simulink model "Car_14DOF_Lat_Long_Control_DATAGEN"  (R2024b)
settings: Solver=ode4  StartTime=0.0  StopTime=30  FixedStep=0.001  RelTol=1e-3
undefined symbols (not defined in the file): Ar1, Ar2, Ar3, Ar4, b, c, C_alpha, C_sigma, f, g, gradbp, Iw, Ix, Iy, Iz, k, ki, kp, kR, L, lf, lh, lr, lw, m, mR, psi0, reff, uFz, x0, xRef2s, y0, yRef2s, z0
libraries: vehdynlibviscommon x1
settings Model: Creator=sherlock2204  LastModifiedBy=sherlock2204

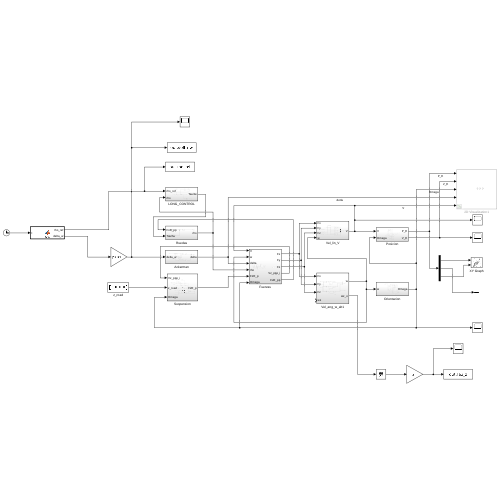
[thumbnail: Simulink's stored preview of the top-level diagram]
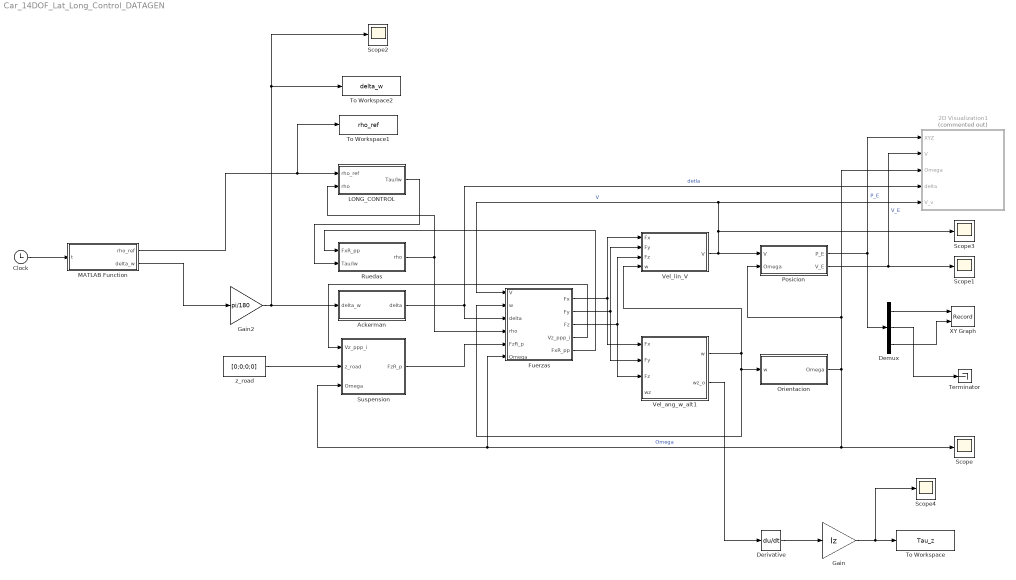
== system Car_14DOF_Lat_Long_Control_DATAGEN ==
  2D Visualization1 : Subsystem  Commented=on
      mask Display: image("visualization.JPG");
  Ackerman : Subsystem
  Clock : Clock
  Demux : Demux  Outputs=3
  Derivative : Derivative
  Fuerzas : Subsystem
  Gain : Gain  Gain=Iz
  Gain2 : Gain  Gain=pi/180
  LONG_CONTROL : Subsystem
  MATLAB Function : MATLAB Function  TreatAsAtomicUnit=on
  Orientacion : Subsystem
  Posicion : Subsystem
  Ruedas : Subsystem
  Scope{,1..4} (5 alike) : Scope
  Suspension : Subsystem
  Terminator : Terminator
  To Workspace : ToWorkspace  VariableName=Tau_z  SaveFormat=Timeseries  SampleTime=-1
  To Workspace1 : ToWorkspace  VariableName=rho_ref  SaveFormat=Timeseries  SampleTime=-1
  To Workspace2 : ToWorkspace  VariableName=delta_w  SaveFormat=Timeseries  SampleTime=-1
  Vel_ang_w_alt1 : Subsystem
  Vel_lin_V : Subsystem
  XY Graph : Record  FileSettingsInternal="{\"entries\":[{\"content\":{\"excelSettings\":{\"content\":{},\"type\":\"Streamout.ExcelSettings\"}},\"type\":\"Streamout.FileSettingStorage\",\"uuid\":\"\"}],\"packageUris\":[\"http:\\/\\/schema.mathworks.com\\/mf0\\/streamout_blocks\\/R2020a\"],\"version\":\"1.0\"}"  Layout=[1 1]  SignalsInternal="{\"entries\":[{\"content\":{\"signals\":[{\"content\":{\"blockPath\":[],\"dimensions\":[1],\"domain\":\"\",\"lineColor\":\"#edb120\",\"lineWidth\":2,\"port\":1,\"sid\":[\"\"],\"signalID\":1,\"signalName\":\"Demux:1\"},\"type\":\"RecordBlkView.Signal\",\"uuid\":\"\"},{\"content\":{\"blockPath\":[],\"dimensions\":[1],\"domain\":\"\",\"lineColor\":\"#7e2f8e\",\"lineWidth\":2,\"port\":2,\"sid\":[\"\"],\"signalID\":2,\"signalName\":\"Demux:3\"},\"type\":\"RecordBlkView.Signal\",\"uuid\":\"\"}]},\"type\":\"RecordBlkView.InputSignals\",\"uuid\":\"\"}],\"packageUris\":[\"http:\\/\\/schema.mathworks.com\\/mf0\\/streamout_blocks\\/R2020a\"],\"version\":\"1.0\"}"  VisualizationBindings="{\"xyplotplugin\":{\"info\":[{\"series\":[],\"subplotID\":1}]}}"  CompatibilityTag=XY
  z_road : Constant  Value=[0;0;0;0]
  wires:
  z_road/1 -> Suspension/2(z_road)
  Fuerzas/3(Fz) -> Vel_ang_w_alt1/3(Fz), Vel_lin_V/3(Fz)
  Vel_ang_w_alt1/1(w) -> Orientacion/1(w), Fuerzas/2(w), Vel_lin_V/4(w)
  Vel_lin_V/1(V) -> Posicion/1(V), Scope3/1, 2D Visualization1/5(V_v), Fuerzas/1(V)  "V"
  Suspension/1(FzR_p) -> Fuerzas/5(FzR_p)
  Fuerzas/4(Vz_ppp_i) -> Suspension/1(Vz_ppp_i)
  Ackerman/1(delta) -> 2D Visualization1/4(delta), Fuerzas/3(delta)  "detla"
  Demux/1 -> XY Graph/1
  Demux/3 -> XY Graph/2
  Demux/2 -> Terminator/1
  Fuerzas/1(Fx) -> Vel_ang_w_alt1/1(Fx), Vel_lin_V/1(Fx)
  Fuerzas/2(Fy) -> Vel_ang_w_alt1/2(Fy), Vel_lin_V/2(Fy)
  Orientacion/1(Omega) -> 2D Visualization1/3(Omega), Posicion/2(Omega), Scope/1, Fuerzas/6(Omega), Suspension/3(Omega)  "Omega"
  Posicion/2(V_E) -> Scope1/1, 2D Visualization1/2(V)  "V_E"
  Posicion/1(P_E) -> Demux/1, 2D Visualization1/1(XYZ)  "P_E"
  Fuerzas/5(FxR_pp) -> Ruedas/1(FxR_pp)
  Ruedas/1(rho) -> Fuerzas/4(rho), LONG_CONTROL/2(rho)
  MATLAB Function/1(rho_ref) -> To Workspace1/1, LONG_CONTROL/1(rho_ref)
  LONG_CONTROL/1(Tau/Iw) -> Ruedas/2(Tau/Iw)
  Gain2/1 -> To Workspace2/1, Scope2/1, Ackerman/1(delta_w)
  Clock/1 -> MATLAB Function/1(t)
  Vel_ang_w_alt1/2(wz_o) -> Derivative/1
  Derivative/1 -> Gain/1
  Gain/1 -> Scope4/1, To Workspace/1
  MATLAB Function/2(delta_w) -> Gain2/1

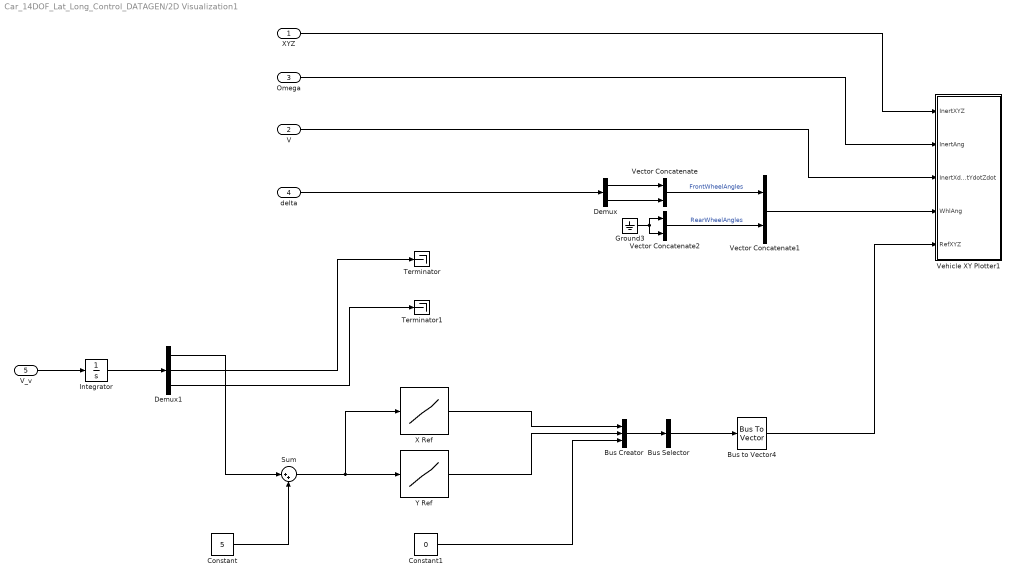
== system Car_14DOF_Lat_Long_Control_DATAGEN/2D Visualization1 ==
  XYZ : Inport
  V : Inport  Port=2
  Omega : Inport  Port=3
  delta : Inport  Port=4
  V_v : Inport  Port=5
  Bus Creator : BusCreator  Inputs=3
  Bus Selector : BusSelector  OutputSignals=signal1,signal2,signal3  OutputAsBus=on
  Bus to Vector4 : BusToVector
  Constant : Constant  Value=5
  Constant1 : Constant  Value=0
  Demux : Demux  Outputs=2
  Demux1 : Demux  Outputs=3
  Ground3 : Ground
  Integrator : Integrator
  Sum : Sum  Inputs=|++
  Terminator : Terminator
  Terminator1 : Terminator
  Vector Concatenate : Concatenate
  Vector Concatenate1 : Concatenate
  Vector Concatenate2 : Concatenate
  Vehicle XY Plotter1 : Subsystem  mask(Vehicle XY Plotter){extRef=on, extStats=off, extTireF=off, a=lf, b=lr, w=c, figBorder=10, bufferSize=1024, velNorm=5, tireFNorm=1000, pltDT=0.2}
      mask prompts: extRef "Plot path reference, extRef"; extStats "Display speed, RPM and Gear"; extTireF "Display tire forces"; a "Distance to front axle from CG, a [m]:"; b "Distance to rear axle from CG, b [m]:"; w "Track width, w [m]:"; figBorder "Distance to figure borders, figBorder [m]:"; bufferSize "Path buffer sampe size, bufferSize []:"; velNorm "Velocity vector scaling, velNorm [m*s/m]:"; tireFNorm "Tire force vector scaling, tireFNorm [m/N]:"; pltDT "Plot update rate, pltDT [s]:"
      mask help:
      | This block will display a MATLAB figure which indicates the vehicle path, current position and heading velocity.
      | An optional path reference is also provided.
      mask init:
      | block = gcb;
      | if autoblkschecksimstopped(block)
      |     ParamNames = {'extRef';'extStats';'extTireF';'extTireF'};
      |     PortNames = {'RefXYZ';'Stats';'TireFx';'TireFy'};
      |     for idx=1:length(PortNames)
      |         InportOption  = {'built-in/Ground', [PortNames{idx}, ' Ground'];...
      |             'built-in/Inport',PortNames{idx}};
      |         if ~strcmp(get_param(block,ParamNames{idx}),'on')
      |             NewBlkHdl = autoblksreplaceblock(block, InportOption, 1);
      |             set_param(NewBlkHdl, 'ShowName', 'off');
      |         else
      |             autoblksreplaceblock(block, InportOption, 2);
      |         end
      |     end
      |     InportNames = {'InertXYZ';'InertAng';'InertXdotYdotZdot';'WhlAng';'RefXYZ';'Stats';'TireFx';'TireFy'};
      |     FoundNames = get_param(find_system(block, 'LookUnderMasks', 'all', 'SearchDepth', 1, 'FollowLinks', 'on', 'BlockType', 'Inport'), 'Name');
      |     [~,PortI] = intersect(InportNames, FoundNames);
      |     PortI = sort(PortI);
      |     for idx = 1:length(PortI)
      |         set_param([block, '/', InportNames{PortI(idx)}], 'Port', num2str(idx));
      |     end
      | end
      mask TypeOptions a: Vehicle XY Plotter/a
      mask TypeOptions b: Vehicle XY Plotter/b
      mask TypeOptions w: Vehicle XY Plotter/w
      mask TypeOptions figBorder: Vehicle XY Plotter/figBorder
      mask TypeOptions bufferSize: Vehicle XY Plotter/bufferSize
      mask TypeOptions velNorm: Vehicle XY Plotter/velNorm
      mask TypeOptions tireFNorm: Vehicle XY Plotter/tireFNorm
      mask DialogControl Container3 Prompt: Plot and Display Options
  X Ref : Lookup_n-D  NumberOfTableDimensions=1  BreakpointsForDimension1=gradbp  Table=xRef2s  InternalRulePriority=Speed  RndMeth=Simplest
  Y Ref : Lookup_n-D  NumberOfTableDimensions=1  BreakpointsForDimension1=gradbp  Table=yRef2s  InternalRulePriority=Speed  RndMeth=Simplest
  wires:
  Omega/1 -> Vehicle XY Plotter1/2(InertAng)
  XYZ/1 -> Vehicle XY Plotter1/1(InertXYZ)
  V/1 -> Vehicle XY Plotter1/3(InertXdotYdotZdot)
  Vector Concatenate2/1 -> Vector Concatenate1/2  "RearWheelAngles"
  Vector Concatenate/1 -> Vector Concatenate1/1  "FrontWheelAngles"
  Ground3/1 -> Vector Concatenate2/2, Vector Concatenate2/1
  Vector Concatenate1/1 -> Vehicle XY Plotter1/4(WhlAng)
  delta/1 -> Demux/1
  Demux/1 -> Vector Concatenate/1
  Demux/2 -> Vector Concatenate/2
  Bus Creator/1 -> Bus Selector/1
  Y Ref/1 -> Bus Creator/2
  Bus Selector/1 -> Bus to Vector4/1
  Demux1/3 -> Terminator1/1
  X Ref/1 -> Bus Creator/1
  Constant1/1 -> Bus Creator/3
  Bus to Vector4/1 -> Vehicle XY Plotter1/5(RefXYZ)
  Demux1/2 -> Terminator/1
  V_v/1 -> Integrator/1
  Integrator/1 -> Demux1/1
  Demux1/1 -> Sum/1
  Sum/1 -> X Ref/1, Y Ref/1
  Constant/1 -> Sum/2

== system Car_14DOF_Lat_Long_Control_DATAGEN/Ackerman ==
  delta_w : Inport
  Atan : Trigonometry  Operator=atan
  Atan1 : Trigonometry  Operator=atan
  Constant : Constant  Value=L
  Divide : Product  Inputs=*/
  Divide1 : Product  Inputs=*/
  Gain : Gain  Gain=L
  Gain1 : Gain  Gain=lw
  Mux : Mux  Inputs=2
  Sum : Sum  Inputs=++|
  Sum1 : Sum  Inputs=-+|
  Tan : Trigonometry  Operator=tan
  delta : Outport
  wires:
  Mux/1 -> delta/1
  delta_w/1 -> Tan/1
  Tan/1 -> Gain/1, Gain1/1
  Gain/1 -> Divide1/1, Divide/1
  Divide/1 -> Atan/1
  Constant/1 -> Sum/2, Sum1/2
  Gain1/1 -> Sum/1, Sum1/1
  Sum/1 -> Divide/2
  Sum1/1 -> Divide1/2
  Divide1/1 -> Atan1/1
  Atan/1 -> Mux/1
  Atan1/1 -> Mux/2

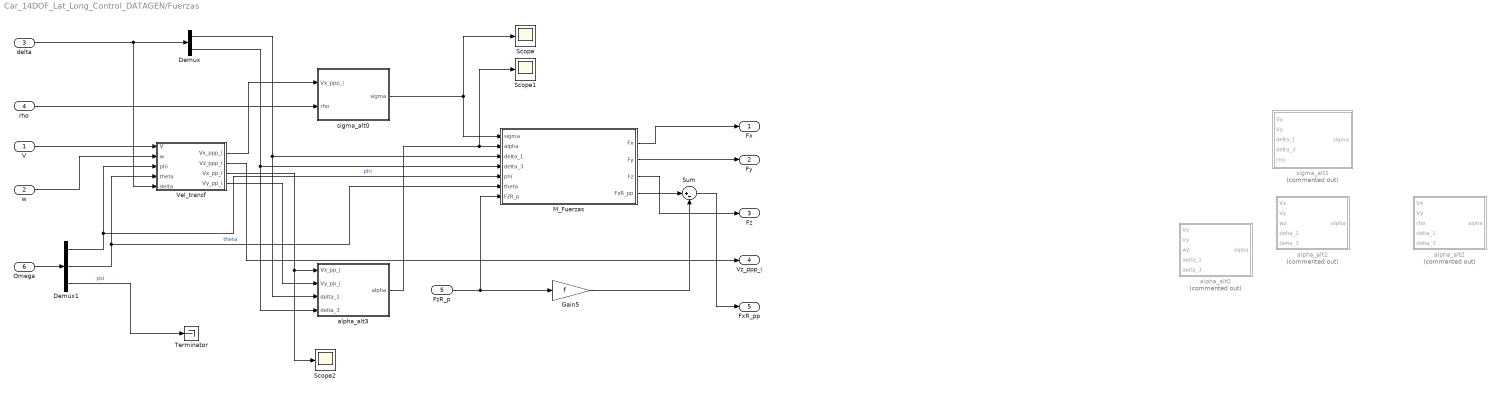
== system Car_14DOF_Lat_Long_Control_DATAGEN/Fuerzas ==
  V : Inport
  w : Inport  Port=2
  delta : Inport  Port=3
  rho : Inport  Port=4
  FzR_p : Inport  Port=5
  Omega : Inport  Port=6
  Demux : Demux  Outputs=2
  Demux1 : Demux  Outputs=3
  Gain5 : Gain  Gain=f
  M_Fuerzas : Subsystem
  Scope : Scope
  Scope1 : Scope
  Scope2 : Scope
  Sum : Sum  Inputs=|+-
  Terminator : Terminator
  Vel_transf : Subsystem
  alpha_alt0 : Subsystem  Commented=on
  alpha_alt1 : Subsystem  Commented=on
  alpha_alt2 : Subsystem  Commented=on
  alpha_alt3 : Subsystem
  sigma_alt0 : Subsystem
  sigma_alt1 : Subsystem  Commented=on
  Fx : Outport
  Fy : Outport  Port=2
  Fz : Outport  Port=3
  Vz_ppp_i : Outport  Port=4
  FxR_pp : Outport  Port=5
  wires:
  V/1 -> Vel_transf/1(V)
  w/1 -> Vel_transf/2(w)
  Demux1/1 -> Vel_transf/3(phi), M_Fuerzas/5(phi)  "phi"
  Demux1/2 -> M_Fuerzas/6(theta), Vel_transf/4(theta)  "theta"
  M_Fuerzas/2(Fy) -> Fy/1
  M_Fuerzas/3(Fz) -> Fz/1
  delta/1 -> Vel_transf/5(delta), Demux/1
  Demux/2 -> alpha_alt3/4(delta_3), M_Fuerzas/4(delta_3)
  Demux/1 -> M_Fuerzas/3(delta_1), alpha_alt3/3(delta_1)
  rho/1 -> sigma_alt0/2(rho)
  Vel_transf/1(Vx_ppp_i) -> sigma_alt0/1(Vx_ppp_i)
  sigma_alt0/1(sigma) -> M_Fuerzas/1(sigma), Scope/1
  alpha_alt3/1(alpha) -> M_Fuerzas/2(alpha), Scope1/1
  FzR_p/1 -> Gain5/1, M_Fuerzas/7(FzR_p)
  Vel_transf/2(Vz_ppp_i) -> Vz_ppp_i/1
  Vel_transf/3(Vx_pp_i) -> Scope2/1, alpha_alt3/1(Vx_pp_i)
  Vel_transf/4(Vy_pp_i) -> alpha_alt3/2(Vy_pp_i)
  Omega/1 -> Demux1/1
  Demux1/3 -> Terminator/1  "psi"
  M_Fuerzas/1(Fx) -> Fx/1
  M_Fuerzas/4(FxR_pp) -> Sum/1
  Sum/1 -> FxR_pp/1
  Gain5/1 -> Sum/2

== system Car_14DOF_Lat_Long_Control_DATAGEN/LONG_CONTROL ==
  rho_ref : Inport
  rho : Inport  Port=2
  Add : Sum  Inputs=+++
  Add1 : Sum  Inputs=++++
  Demux : Demux
  Derivative : Derivative
  Gain : Gain  Gain=[1;1;1;1]
  Gain1 : Gain  Gain=Iw
  Gain2 : Gain  Gain=-ki
  Gain3 : Gain  Gain=-kp
  Integrator5 : Integrator
  Scope : Scope
  Scope1 : Scope
  Sum1 : Sum  Inputs=|-+
  Tau/Iw : Outport
  wires:
  Gain/1 -> Sum1/1, Derivative/1
  Add/1 -> Gain1/1, Tau/Iw/1  "u=Tau/Iw"
  Integrator5/1 -> Gain2/1  "Ie_rho"
  Gain3/1 -> Add/2
  Sum1/1 -> Integrator5/1, Gain3/1  "e_rho"
  Gain2/1 -> Add/1  "-z"
  Derivative/1 -> Add/3  "Drho_ref"
  rho_ref/1 -> Gain/1
  rho/1 -> Scope1/1, Sum1/2
  Gain1/1 -> Demux/1
  Demux/1 -> Add1/1
  Demux/2 -> Add1/2
  Demux/3 -> Add1/3
  Demux/4 -> Add1/4
  Add1/1 -> Scope/1

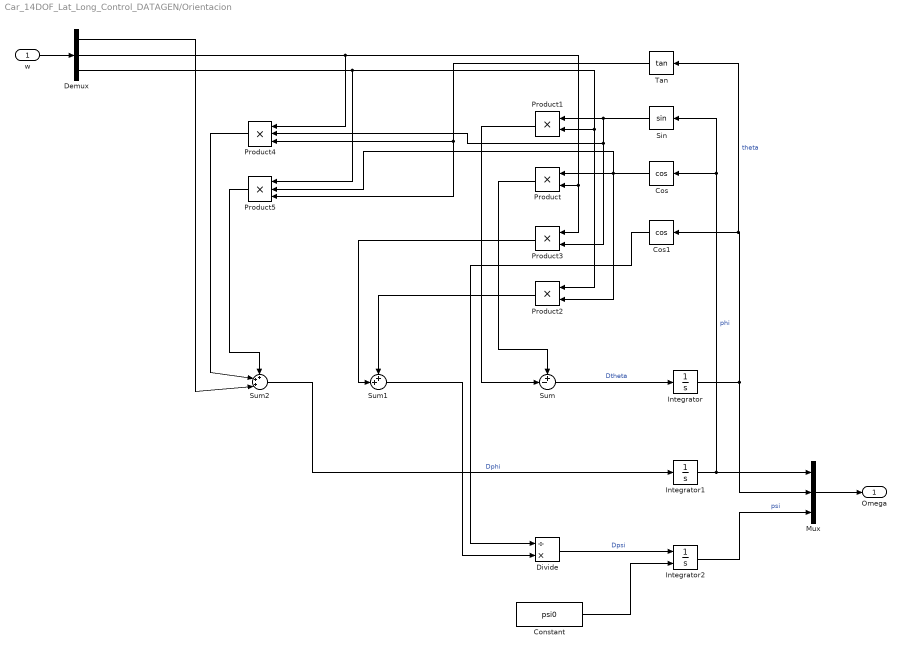
== system Car_14DOF_Lat_Long_Control_DATAGEN/Orientacion ==
  w : Inport
  Constant : Constant  Value=psi0
  Cos : Trigonometry  Operator=cos
  Cos1 : Trigonometry  Operator=cos
  Demux : Demux  Outputs=3
  Divide : Product  Inputs=/*
  Integrator : Integrator
  Integrator1 : Integrator
  Integrator2 : Integrator  InitialConditionSource=external
  Mux : Mux  Inputs=3
  Product{,1..3} (4 alike) : Product
  Product4 : Product  Inputs=3
  Product5 : Product  Inputs=3
  Sin : Trigonometry
  Sum : Sum  Inputs=+-|
  Sum1 : Sum  Inputs=++|
  Sum2 : Sum  Inputs=+++|
  Tan : Trigonometry  Operator=tan
  Omega : Outport
  wires:
  w/1 -> Demux/1
  Integrator/1 -> Mux/2, Tan/1, Cos1/1  "theta"
  Integrator2/1 -> Mux/3  "psi"
  Sin/1 -> Product4/2, Product3/2, Product1/1
  Cos/1 -> Product5/2, Product2/2, Product/1
  Demux/2 -> Product4/1, Product3/1, Product/2
  Demux/3 -> Product5/1, Product2/1, Product1/2
  Product/1 -> Sum/1
  Product1/1 -> Sum/2
  Sum/1 -> Integrator/1  "Dtheta"
  Integrator1/1 -> Sin/1, Cos/1, Mux/1  "phi"
  Product2/1 -> Sum1/1
  Product3/1 -> Sum1/2
  Divide/1 -> Integrator2/1  "Dpsi"
  Sum1/1 -> Divide/2
  Cos1/1 -> Divide/1
  Tan/1 -> Product4/3, Product5/3
  Sum2/1 -> Integrator1/1  "Dphi"
  Product5/1 -> Sum2/1
  Product4/1 -> Sum2/2
  Demux/1 -> Sum2/3
  Mux/1 -> Omega/1
  Constant/1 -> Integrator2/2

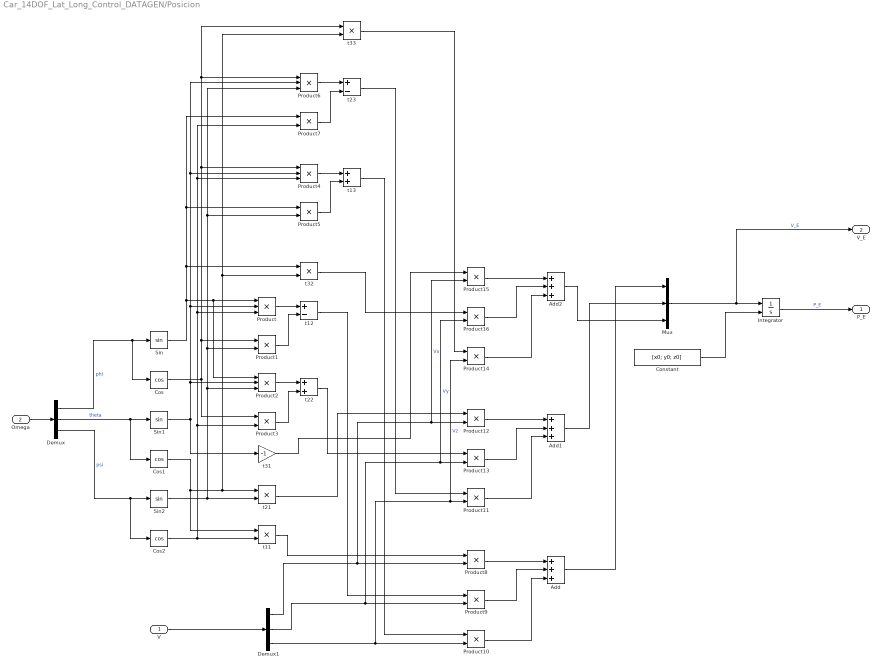
== system Car_14DOF_Lat_Long_Control_DATAGEN/Posicion ==
  V : Inport
  Omega : Inport  Port=2
  Add : Sum  Inputs=+++
  Add1 : Sum  Inputs=+++
  Add2 : Sum  Inputs=+++
  Constant : Constant  Value=[x0; y0; z0]
  Cos : Trigonometry  Operator=cos
  Cos1 : Trigonometry  Operator=cos
  Cos2 : Trigonometry  Operator=cos
  Demux : Demux  Outputs=3
  Demux1 : Demux  Outputs=3
  Integrator : Integrator  InitialConditionSource=external
  Mux : Mux  Inputs=3
  Product{,2,4,6} (4 alike) : Product  Inputs=3
  Product{1,3,5,7..16} (13 alike) : Product
  Sin : Trigonometry
  Sin1 : Trigonometry
  Sin2 : Trigonometry
  t{11,21,32..33} (4 alike) : Product
  t12 : Sum  Inputs=+-
  t13 : Sum
  t22 : Sum
  t23 : Sum  Inputs=+-
  t31 : Gain  Gain=-1
  P_E : Outport
  V_E : Outport  Port=2
  wires:
  Demux/1 -> Cos/1, Sin/1  "phi"
  Demux/2 -> Cos1/1, Sin1/1  "theta"
  Demux/3 -> Cos2/1, Sin2/1  "psi"
  Omega/1 -> Demux/1
  Cos2/1 -> Product7/2, Product4/3, Product/3, Product3/2, t11/2
  Cos1/1 -> t21/1, t33/2, t32/2, t11/1
  Sin2/1 -> Product6/3, Product5/2, Product1/2, Product2/3, t21/2
  Sin1/1 -> Product6/2, Product4/2, Product/2, Product2/2, t31/1
  Sin/1 -> Product7/1, Product5/1, t32/1, Product2/1, Product/1
  Cos/1 -> t33/1, Product6/1, Product4/1, Product1/1, Product3/1
  Product/1 -> t12/1
  Product1/1 -> t12/2
  Product3/1 -> t22/2
  Product2/1 -> t22/1
  Product5/1 -> t13/2
  Product4/1 -> t13/1
  Product6/1 -> t23/1
  Product7/1 -> t23/2
  V/1 -> Demux1/1
  Demux1/1 -> Product15/2, Product12/2, Product8/2  "Vx"
  Demux1/3 -> Product10/2, Product14/2, Product11/2  "Vz"
  Demux1/2 -> Product9/2, Product16/2, Product13/2  "Vy"
  t11/1 -> Product8/1
  t12/1 -> Product9/1
  t13/1 -> Product10/1
  Product8/1 -> Add/1
  Product9/1 -> Add/2
  Product10/1 -> Add/3
  Product13/1 -> Add1/2
  Product12/1 -> Add1/1
  Product11/1 -> Add1/3
  t21/1 -> Product12/1
  t22/1 -> Product13/1
  t23/1 -> Product11/1
  Product15/1 -> Add2/1
  Product16/1 -> Add2/2
  Product14/1 -> Add2/3
  t31/1 -> Product15/1
  t32/1 -> Product16/1
  t33/1 -> Product14/1
  Add/1 -> Mux/1
  Add1/1 -> Mux/2
  Add2/1 -> Mux/3
  Mux/1 -> V_E/1, Integrator/1  "V_E"
  Integrator/1 -> P_E/1  "P_E"
  Constant/1 -> Integrator/2

== system Car_14DOF_Lat_Long_Control_DATAGEN/Ruedas ==
  FxR_pp : Inport
  Tau/Iw : Inport  Port=2
  Gain : Gain  Gain=1/Iw
  Gain13 : Gain  Gain=-reff/Iw
  Integrator4 : Integrator
  Sum : Sum  Inputs=|++
  rho : Outport
  wires:
  FxR_pp/1 -> Gain13/1
  Tau/Iw/1 -> Gain/1  "u=Tau/Iw"
  Sum/1 -> Integrator4/1  "Drho"
  Integrator4/1 -> rho/1
  Gain13/1 -> Sum/2  "EPS(t)"
  Gain/1 -> Sum/1  "Tau"

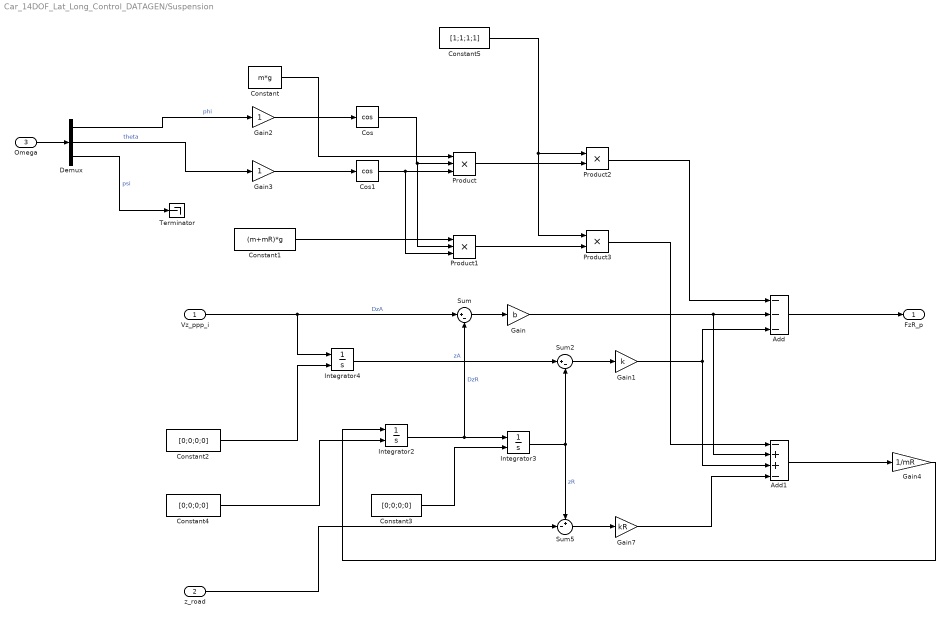
== system Car_14DOF_Lat_Long_Control_DATAGEN/Suspension ==
  Vz_ppp_i : Inport
  z_road : Inport  Port=2
  Omega : Inport  Port=3
  Add : Sum  Inputs=---
  Add1 : Sum  Inputs=-++-
  Constant : Constant  Value=m*g
  Constant1 : Constant  Value=(m+mR)*g
  Constant2 : Constant  Value=[0;0;0;0]
  Constant3 : Constant  Value=[0;0;0;0]
  Constant4 : Constant  Value=[0;0;0;0]
  Constant5 : Constant  Value=[1;1;1;1]
  Cos : Trigonometry  Operator=cos
  Cos1 : Trigonometry  Operator=cos
  Demux : Demux  Outputs=3
  Gain : Gain  Gain=b
  Gain1 : Gain  Gain=k
  Gain2 : Gain
  Gain3 : Gain
  Gain4 : Gain  Gain=1/mR
  Gain7 : Gain  Gain=kR
  Integrator2 : Integrator  InitialConditionSource=external
  Integrator3 : Integrator  InitialConditionSource=external
  Integrator4 : Integrator  InitialConditionSource=external
  Product : Product  Inputs=3
  Product1 : Product  Inputs=3
  Product2 : Product
  Product3 : Product
  Sum : Sum  Inputs=|+-
  Sum2 : Sum  Inputs=|+-
  Sum5 : Sum  Inputs=+-|
  Terminator : Terminator
  FzR_p : Outport
  wires:
  Sum/1 -> Gain/1
  Integrator3/1 -> Sum2/2, Sum5/1  "zR"
  Sum2/1 -> Gain1/1
  Add/1 -> FzR_p/1
  Add1/1 -> Gain4/1
  Gain/1 -> Add1/2, Add/2
  Integrator2/1 -> Integrator3/1, Sum/2  "DzR"
  Gain1/1 -> Add/3, Add1/3
  Sum5/1 -> Gain7/1
  Gain7/1 -> Add1/4
  Gain4/1 -> Integrator2/1
  Constant4/1 -> Integrator2/2
  Constant3/1 -> Integrator3/2
  z_road/1 -> Sum5/2
  Cos1/1 -> Product1/3, Product/3
  Cos/1 -> Product1/2, Product/2
  Constant/1 -> Product/1
  Constant1/1 -> Product1/1
  Vz_ppp_i/1 -> Integrator4/1, Sum/1  "DzA"
  Integrator4/1 -> Sum2/1  "zA"
  Constant2/1 -> Integrator4/2
  Product/1 -> Product2/2
  Constant5/1 -> Product3/1, Product2/1
  Product1/1 -> Product3/2
  Demux/1 -> Gain2/1  "phi"
  Demux/2 -> Gain3/1  "theta"
  Product2/1 -> Add/1
  Product3/1 -> Add1/1
  Gain2/1 -> Cos/1
  Gain3/1 -> Cos1/1
  Omega/1 -> Demux/1
  Demux/3 -> Terminator/1  "psi"

== system Car_14DOF_Lat_Long_Control_DATAGEN/Vel_ang_w_alt1 ==
  Fx : Inport
  Fy : Inport  Port=2
  Fz : Inport  Port=3
  wz : Inport  Port=4
  Integrator : Integrator  InitialConditionSource=external
  Integrator1 : Integrator  InitialConditionSource=external
  Integrator2 : Integrator  InitialConditionSource=external
  Multiply : Gain  Gain=(1/Ix)*[c c -c -c lh lh lh lh]  Multiplication=Matrix(K*u) (u vector)
  Multiply1 : Gain  Gain=(1/Iy)*[-lh -lh -lh -lh -lf lr -lf lr]  Multiplication=Matrix(K*u) (u vector)
  Multiply2 : Gain  Gain=(1/Iz)*[lf -lr lf -lr -c -c c c]  Multiplication=Matrix(K*u) (u vector)
  Mux : Mux  Inputs=3
  Vector Concatenate : Concatenate
  Vector Concatenate1 : Concatenate
  Vector Concatenate2 : Concatenate
  wx0 : Constant  Value=0
  wy0 : Constant  Value=0
  wz0 : Constant  Value=0
  w : Outport
  wz_o : Outport  Port=2
  wires:
  wx0/1 -> Integrator/2
  wy0/1 -> Integrator1/2
  Mux/1 -> w/1
  wz0/1 -> Integrator2/2
  Integrator/1 -> Mux/1  "wx"
  Fz/1 -> Vector Concatenate/1, Vector Concatenate1/2
  Fy/1 -> Vector Concatenate/2, Vector Concatenate2/1
  Vector Concatenate/1 -> Multiply/1
  Multiply1/1 -> Integrator1/1
  Vector Concatenate1/1 -> Multiply1/1
  Fx/1 -> Vector Concatenate2/2, Vector Concatenate1/1
  Integrator1/1 -> Mux/2  "wy"
  Vector Concatenate2/1 -> Multiply2/1
  Integrator2/1 -> Mux/3, wz_o/1  "wz"
  Multiply/1 -> Integrator/1
  Multiply2/1 -> Integrator2/1

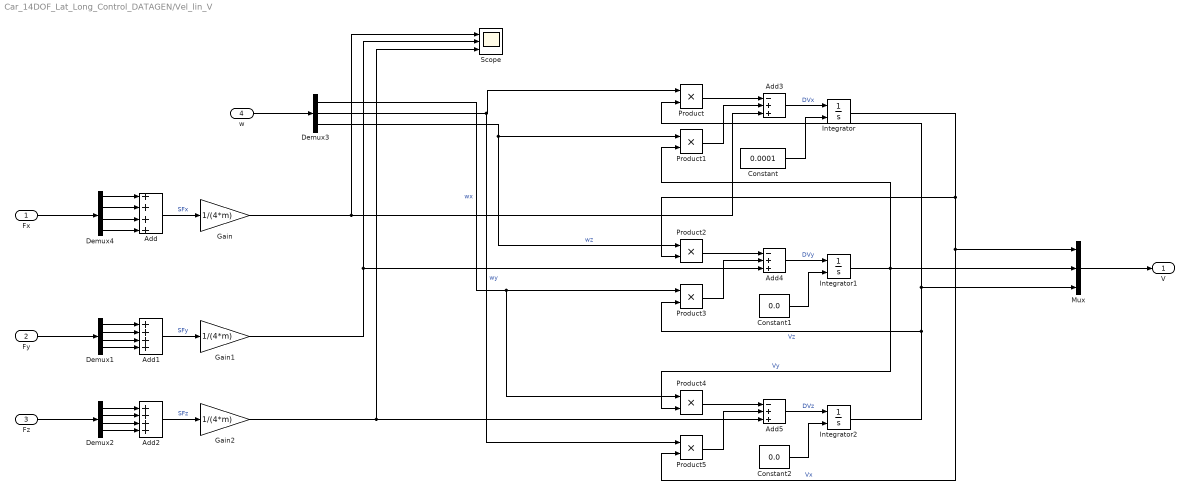
== system Car_14DOF_Lat_Long_Control_DATAGEN/Vel_lin_V ==
  Fx : Inport
  Fy : Inport  Port=2
  Fz : Inport  Port=3
  w : Inport  Port=4
  Add : Sum  Inputs=++++
  Add1 : Sum  Inputs=++++
  Add2 : Sum  Inputs=++++
  Add3 : Sum  Inputs=-++
  Add4 : Sum  Inputs=-++
  Add5 : Sum  Inputs=-++
  Constant : Constant  Value=0.0001  SampleTime=0.001
  Constant1 : Constant  Value=0.0
  Constant2 : Constant  Value=0.0
  Demux1 : Demux
  Demux2 : Demux
  Demux3 : Demux  Outputs=3
  Demux4 : Demux
  Gain : Gain  Gain=1/(4*m)
  Gain1 : Gain  Gain=1/(4*m)
  Gain2 : Gain  Gain=1/(4*m)
  Integrator : Integrator  InitialConditionSource=external  UpperSaturationLimit=27.7778  LowerSaturationLimit=-27.7778  AbsoluteTolerance=10
  Integrator1 : Integrator  InitialConditionSource=external
  Integrator2 : Integrator  InitialConditionSource=external
  Mux : Mux  Inputs=3
  Product{,1..5} (6 alike) : Product
  Scope : Scope  NumInputPorts=3
  V : Outport
  wires:
  Fy/1 -> Demux1/1
  Demux1/1 -> Add1/1
  Demux1/2 -> Add1/2
  Demux1/3 -> Add1/3
  Demux1/4 -> Add1/4
  Demux2/1 -> Add2/1
  Fz/1 -> Demux2/1
  Demux2/2 -> Add2/2
  Demux2/4 -> Add2/4
  Demux2/3 -> Add2/3
  w/1 -> Demux3/1
  Add/1 -> Gain/1  "SFx"
  Add1/1 -> Gain1/1  "SFy"
  Add2/1 -> Gain2/1  "SFz"
  Add3/1 -> Integrator/1  "DVx"
  Product1/1 -> Add3/2
  Product/1 -> Add3/1
  Demux3/3 -> Product2/1, Product1/1  "wz"
  Demux3/2 -> Product5/1, Product/1  "wy"
  Product2/1 -> Add4/1
  Add4/1 -> Integrator1/1  "DVy"
  Product3/1 -> Add4/2
  Add5/1 -> Integrator2/1  "DVz"
  Product4/1 -> Add5/1
  Product5/1 -> Add5/2
  Demux3/1 -> Product4/1, Product3/1  "wx"
  Integrator1/1 -> Mux/2, Product1/2, Product4/2  "Vy"
  Integrator2/1 -> Product3/2, Mux/3, Product/2  "Vz"
  Integrator/1 -> Mux/1, Product5/2, Product2/2  "Vx"
  Mux/1 -> V/1
  Demux4/1 -> Add/1
  Demux4/4 -> Add/4
  Demux4/2 -> Add/2
  Demux4/3 -> Add/3
  Fx/1 -> Demux4/1
  Constant/1 -> Integrator/2
  Constant1/1 -> Integrator1/2
  Constant2/1 -> Integrator2/2
  Gain/1 -> Scope/1, Add3/3
  Gain1/1 -> Scope/2, Add4/3
  Gain2/1 -> Scope/3, Add5/3

== system Car_14DOF_Lat_Long_Control_DATAGEN/2D Visualization1/Vehicle XY Plotter1 ==
  InertXYZ : Inport
  InertAng : Inport  Port=2
  InertXdotYdotZdot : Inport  Port=3
  WhlAng : Inport  Port=4
  RefXYZ : Inport  Port=5
  Data Type Conversion : DataTypeConversion  OutDataTypeStr=double  SaturateOnIntegerOverflow=off  RndMeth=Floor
  Rate Transition{1..7} (7 alike) : RateTransition  Deterministic=off  OutPortSampleTime=pltDT
  Reshape : Reshape  OutputDimensionality=Row vector (2-D)
  Reshape1 : Reshape  OutputDimensionality=Row vector (2-D)
  Stats Ground : Ground
  TireFx Ground : Ground
  TireFy Ground : Ground
  Vector Concatenate : Concatenate  Mode=Multidimensional array
  Vehicle XY Plotter : vehdynlibviscommon/Vehicle XY Plotter  w=w  a=a  b=b  figBorder=figBorder  bufferSize=bufferSize  extStats=off  extTireF=off
  wires:
  Stats Ground/1 -> Data Type Conversion/1
  InertAng/1 -> Rate Transition2/1  "InertCGDisp"
  InertXdotYdotZdot/1 -> Rate Transition4/1  "InertCGVel"
  InertXYZ/1 -> Rate Transition1/1  "InertCGDisp"
  WhlAng/1 -> Rate Transition5/1  "WhlAng"
  Rate Transition3/1 -> Vehicle XY Plotter/5
  Rate Transition1/1 -> Vehicle XY Plotter/1
  Rate Transition2/1 -> Vehicle XY Plotter/2
  Rate Transition4/1 -> Vehicle XY Plotter/3
  Rate Transition5/1 -> Vehicle XY Plotter/4
  Rate Transition6/1 -> ?
  Data Type Conversion/1 -> Rate Transition6/1
  Rate Transition7/1 -> ?
  Reshape/1 -> Vector Concatenate/1
  Reshape1/1 -> Vector Concatenate/2
  Vector Concatenate/1 -> Rate Transition7/1
  TireFx Ground/1 -> Reshape/1
  TireFy Ground/1 -> Reshape1/1
  RefXYZ/1 -> Rate Transition3/1

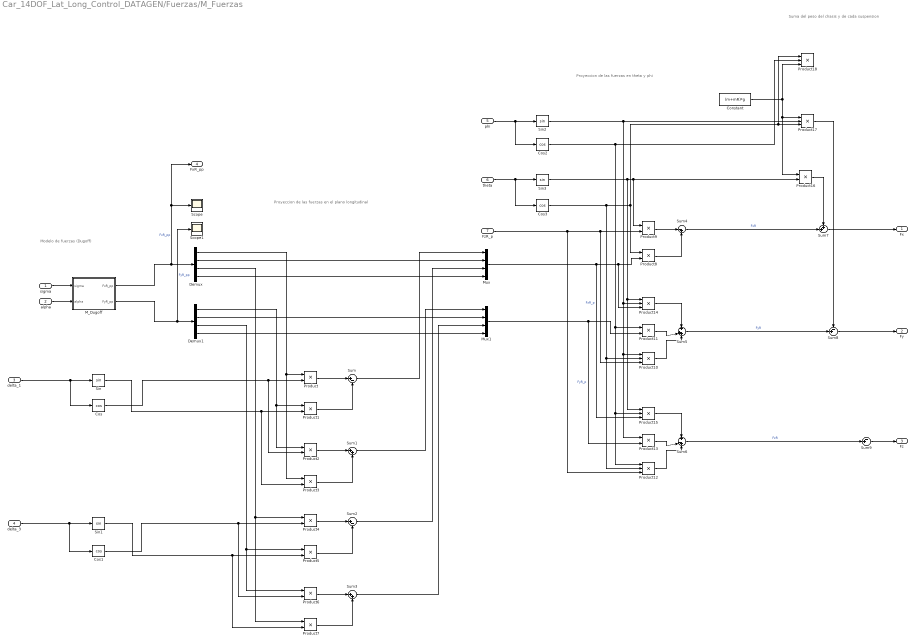
== system Car_14DOF_Lat_Long_Control_DATAGEN/Fuerzas/M_Fuerzas ==
  note: Modelo de fuerzas (Dugoff)
  note: Suma del peso del chasis
      | y de cada suspension
  note: Proyeccion de las fuerzas en theta y phi
  note: Proyeccion de las fuerzas en el plano longitudinal
  sigma : Inport
  alpha : Inport  Port=2
  delta_1 : Inport  Port=3
  delta_3 : Inport  Port=4
  phi : Inport  Port=5
  theta : Inport  Port=6
  FzR_p : Inport  Port=7
  Constant : Constant  Value=(m+mR)*g
  Cos{,1..3} (4 alike) : Trigonometry  Operator=cos
  Demux : Demux
  Demux1 : Demux
  M_Dugoff : Subsystem
  Mux : Mux
  Mux1 : Mux
  Product{,1..9,11,13,16} (13 alike) : Product
  Product{10,12,14..15,17..18} (6 alike) : Product  Inputs=3
  Scope : Scope
  Scope1 : Scope
  Sin{,1..3} (4 alike) : Trigonometry
  Sum : Sum  Inputs=|+-
  Sum1 : Sum  Inputs=|++
  Sum2 : Sum  Inputs=|+-
  Sum3 : Sum  Inputs=|++
  Sum4 : Sum  Inputs=|-+
  Sum5 : Sum  Inputs=+|++
  Sum6 : Sum  Inputs=+|-+
  Sum7 : Sum  Inputs=++|
  Sum8 : Sum  Inputs=-+|
  Sum9 : Sum  Inputs=-+|
  Fx : Outport
  Fy : Outport  Port=2
  Fz : Outport  Port=3
  FxR_pp : Outport  Port=4
  wires:
  M_Dugoff/2(FyR_pp) -> Scope1/1, Demux1/1  "FyR_pp"
  Demux/2 -> Mux/2
  Demux/4 -> Mux/4
  Demux1/2 -> Mux1/2
  Demux1/4 -> Mux1/4
  Demux/1 -> Product3/1, Product/1
  Cos/1 -> Product2/2, Product/2
  Product/1 -> Sum/1
  Sin/1 -> Product3/2, Product1/2
  Demux1/1 -> Product2/1, Product1/1
  Product1/1 -> Sum/2
  Sum/1 -> Mux/1
  Product2/1 -> Sum1/1
  Product3/1 -> Sum1/2
  Sum1/1 -> Mux1/1
  Product6/1 -> Sum3/1
  Product7/1 -> Sum3/2
  Product5/1 -> Sum2/2
  Product4/1 -> Sum2/1
  Demux/3 -> Product7/1, Product4/1
  Demux1/3 -> Product6/1, Product5/1
  Cos1/1 -> Product6/2, Product4/2
  Sin1/1 -> Product7/2, Product5/2
  Sum2/1 -> Mux/3
  Sum3/1 -> Mux1/3
  Mux/1 -> Product15/3, Product14/3, Product8/2  "FxR_p"
  FzR_p/1 -> Product12/3, Product9/2, Product10/3
  Cos3/1 -> Product12/2, Product10/2, Product18/1, Product17/3, Product8/1
  Sin3/1 -> Product15/1, Product14/1, Product9/1, Product16/2
  Product9/1 -> Sum4/1
  Product8/1 -> Sum4/2
  Product10/1 -> Sum5/3
  Sum5/1 -> Sum8/2  "FyR"
  Product11/1 -> Sum5/2
  Product13/1 -> Sum6/2
  Product12/1 -> Sum6/3
  Sum6/1 -> Sum9/2  "FzR"
  Product14/1 -> Sum5/1
  Sin2/1 -> Product17/2, Product13/1, Product10/1, Product14/2
  Mux1/1 -> Product11/2, Product13/2  "FyR_p"
  Cos2/1 -> Product18/2, Product11/1, Product12/1, Product15/2
  Product15/1 -> Sum6/1
  Constant/1 -> Product18/3, Product16/1, Product17/1
  Sum4/1 -> Sum7/2  "FxR"
  Sum7/1 -> Fx/1
  Product16/1 -> Sum7/1
  Sum8/1 -> Fy/1
  Product17/1 -> Sum8/1
  sigma/1 -> M_Dugoff/1(sigma)
  alpha/1 -> M_Dugoff/2(alpha)
  M_Dugoff/1(FxR_pp) -> Scope/1, FxR_pp/1, Demux/1  "FxR_pp"
  Sum9/1 -> Fz/1
  phi/1 -> Cos2/1, Sin2/1
  theta/1 -> Cos3/1, Sin3/1
  delta_1/1 -> Cos/1, Sin/1
  delta_3/1 -> Cos1/1, Sin1/1

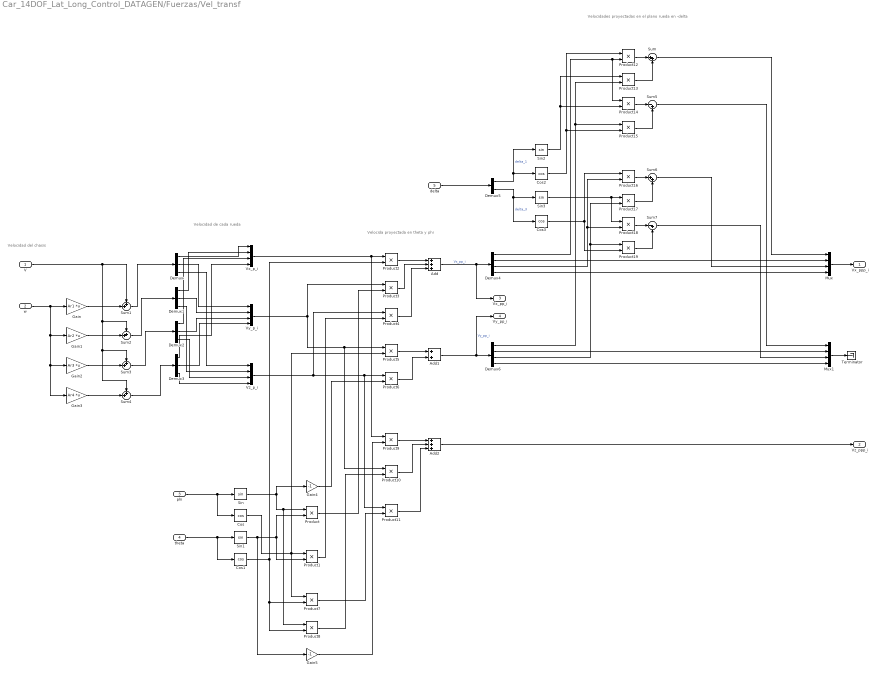
== system Car_14DOF_Lat_Long_Control_DATAGEN/Fuerzas/Vel_transf ==
  note: Velocidades proyectadas en el plano rueda en -delta
  note: Velocida proyectada en theta y phi
  note: Velocidad de cada rueda
  note: Velocidad del chasis
  V : Inport
  w : Inport  Port=2
  phi : Inport  Port=3
  theta : Inport  Port=4
  delta : Inport  Port=5
  Add : Sum  Inputs=+++
  Add1 : Sum
  Add2 : Sum  Inputs=+++
  Cos{,1..3} (4 alike) : Trigonometry  Operator=cos
  Demux{,1..3} (4 alike) : Demux  Outputs=3
  Demux4 : Demux
  Demux5 : Demux  Outputs=2
  Demux6 : Demux
  Gain : Gain  Gain=Ar1  Multiplication=Matrix(K*u)
  Gain1 : Gain  Gain=Ar2  Multiplication=Matrix(K*u)
  Gain2 : Gain  Gain=Ar3  Multiplication=Matrix(K*u)
  Gain3 : Gain  Gain=Ar4  Multiplication=Matrix(K*u)
  Gain4 : Gain  Gain=-1
  Gain5 : Gain  Gain=-1
  Mux : Mux
  Mux1 : Mux
  Product{,1..19} (20 alike) : Product
  Sin{,1..3} (4 alike) : Trigonometry
  Sum : Sum  Inputs=|++
  Sum{1..4} (4 alike) : Sum  Inputs=++|
  Sum5 : Sum  Inputs=|-+
  Sum6 : Sum  Inputs=|++
  Sum7 : Sum  Inputs=|-+
  Terminator : Terminator
  Vx_p_i : Mux
  Vy_p_i : Mux
  Vz_p_i : Mux
  Vx_ppp_i : Outport
  Vz_ppp_i : Outport  Port=2
  Vx_pp_i : Outport  Port=3
  Vy_pp_i : Outport  Port=4
  wires:
  w/1 -> Gain3/1, Gain2/1, Gain1/1, Gain/1
  Gain/1 -> Sum1/2
  Gain1/1 -> Sum2/2
  V/1 -> Sum2/1, Sum4/1, Sum3/1, Sum1/1
  Gain2/1 -> Sum3/2
  Gain3/1 -> Sum4/2
  Sum1/1 -> Demux/1
  Sum2/1 -> Demux1/1
  Sum3/1 -> Demux2/1
  Sum4/1 -> Demux3/1
  Demux/1 -> Vx_p_i/1
  Demux1/1 -> Vx_p_i/2
  Demux2/1 -> Vx_p_i/3
  Demux3/1 -> Vx_p_i/4
  Demux/2 -> Vy_p_i/1
  Demux1/2 -> Vy_p_i/2
  Demux2/2 -> Vy_p_i/3
  Demux3/2 -> Vy_p_i/4
  Demux/3 -> Vz_p_i/1
  Demux1/3 -> Vz_p_i/2
  Demux2/3 -> Vz_p_i/3
  Demux3/3 -> Vz_p_i/4
  Sin1/1 -> Gain5/1, Product1/2, Product/2
  Cos/1 -> Product7/1, Product1/1, Product5/2
  Sin/1 -> Gain4/1, Product8/1, Product/1
  Vx_p_i/1 -> Product9/1, Product2/1
  Cos1/1 -> Product8/2, Product7/2, Product2/2
  Product2/1 -> Add/1
  Product3/1 -> Add/2
  Product/1 -> Product3/2
  Vy_p_i/1 -> Product10/1, Product5/1, Product3/1
  Vz_p_i/1 -> Product4/1, Product11/1, Product6/1
  Product1/1 -> Product4/2
  Product4/1 -> Add/3
  Product5/1 -> Add1/1
  Gain4/1 -> Product6/2
  Product6/1 -> Add1/2
  Add2/1 -> Vz_ppp_i/1
  Product9/1 -> Add2/1
  Gain5/1 -> Product9/2
  Product10/1 -> Add2/2
  Product8/1 -> Product10/2
  Product11/1 -> Add2/3
  Product7/1 -> Product11/2
  Add/1 -> Vx_pp_i/1, Demux4/1  "Vx_pp_i"
  Add1/1 -> Vy_pp_i/1, Demux6/1  "Vy_pp_i"
  Mux/1 -> Vx_ppp_i/1
  Demux4/2 -> Mux/2
  Demux4/4 -> Mux/4
  Demux6/2 -> Mux1/2
  Demux6/4 -> Mux1/4
  Demux5/1 -> Cos2/1, Sin2/1  "delta_1"
  Demux5/2 -> Sin3/1, Cos3/1  "delta_3"
  Cos2/1 -> Product15/2, Product12/1
  Product12/1 -> Sum/1
  Product13/1 -> Sum/2
  Product14/1 -> Sum5/1
  Product15/1 -> Sum5/2
  Sin2/1 -> Product14/2, Product13/1
  Product16/1 -> Sum6/1
  Product17/1 -> Sum6/2
  Product19/1 -> Sum7/2
  Product18/1 -> Sum7/1
  Demux4/1 -> Product12/2, Product14/1
  Demux6/1 -> Product13/2, Product15/1
  Sum/1 -> Mux/1
  Sum5/1 -> Mux1/1
  Cos3/1 -> Product19/2, Product16/1
  Demux4/3 -> Product18/2, Product16/2
  Demux6/3 -> Product19/1, Product17/2
  Sin3/1 -> Product18/1, Product17/1
  Sum6/1 -> Mux/3
  Sum7/1 -> Mux1/3
  Mux1/1 -> Terminator/1
  phi/1 -> Cos/1, Sin/1
  theta/1 -> Cos1/1, Sin1/1
  delta/1 -> Demux5/1

== system Car_14DOF_Lat_Long_Control_DATAGEN/Fuerzas/alpha_alt0 ==
  Vx : Inport
  Vy : Inport  Port=2
  wz : Inport  Port=3
  delta_1 : Inport  Port=4
  delta_3 : Inport  Port=5
  Atan : Trigonometry  Operator=atan
  Atan1 : Trigonometry  Operator=atan
  Divide : Product  Inputs=/*
  Divide1 : Product  Inputs=/*
  Gain : Gain  Gain=lf
  Gain1 : Gain  Gain=lr
  Gain2 : Gain  Gain=-1
  Mux : Mux
  Sum : Sum  Inputs=+-|
  Sum1 : Sum  Inputs=++|
  Sum2 : Sum  Inputs=|-+
  Sum3 : Sum  Inputs=-+|
  alpha : Outport
  wires:
  wz/1 -> Gain/1, Gain1/1
  Vy/1 -> Sum1/1, Sum/1
  Sum/1 -> Divide/2
  Vx/1 -> Divide1/1, Divide/1
  Divide/1 -> Atan/1
  Atan/1 -> Gain2/1
  Gain2/1 -> Mux/4, Mux/2
  Sum1/1 -> Divide1/2
  Divide1/1 -> Atan1/1
  Atan1/1 -> Sum3/1, Sum2/1
  delta_1/1 -> Sum2/2
  Sum2/1 -> Mux/1
  delta_3/1 -> Sum3/2
  Sum3/1 -> Mux/3
  Mux/1 -> alpha/1

== system Car_14DOF_Lat_Long_Control_DATAGEN/Fuerzas/alpha_alt1 ==
  Vx : Inport
  Vy : Inport  Port=2
  wz : Inport  Port=3
  delta_1 : Inport  Port=4
  delta_3 : Inport  Port=5
  Atan : Trigonometry  Operator=atan
  Atan1 : Trigonometry  Operator=atan
  Divide : Product  Inputs=/*
  Divide1 : Product  Inputs=/*
  Gain : Gain  Gain=lf
  Gain1 : Gain  Gain=lr
  Gain2 : Gain  Gain=-1
  Mux : Mux
  Sum : Sum  Inputs=+-|
  Sum1 : Sum  Inputs=++|
  Sum2 : Sum  Inputs=|-+
  Sum3 : Sum  Inputs=+-|
  alpha : Outport
  wires:
  wz/1 -> Gain/1, Gain1/1
  Vy/1 -> Sum1/1, Sum/1
  Sum/1 -> Divide/2
  Vx/1 -> Divide1/1, Divide/1
  Divide/1 -> Atan/1
  Atan/1 -> Gain2/1
  Gain2/1 -> Mux/4, Mux/2
  Sum1/1 -> Divide1/2
  Divide1/1 -> Atan1/1
  Atan1/1 -> Sum3/1, Sum2/1
  delta_1/1 -> Sum2/2
  Sum2/1 -> Mux/1
  delta_3/1 -> Sum3/2
  Sum3/1 -> Mux/3
  Mux/1 -> alpha/1

== system Car_14DOF_Lat_Long_Control_DATAGEN/Fuerzas/alpha_alt2 ==
  Vx : Inport
  Vy : Inport  Port=2
  rho : Inport  Port=3
  delta_1 : Inport  Port=4
  delta_3 : Inport  Port=5
  Abs : Abs  SaturateOnIntegerOverflow=off
  Abs1 : Abs  SaturateOnIntegerOverflow=off
  Atan : Trigonometry  Operator=atan
  Atan1 : Trigonometry  Operator=atan
  Demux : Demux
  Divide : Product  Inputs=/*
  Divide1 : Product  Inputs=/*
  Gain : Gain  Gain=reff
  Gain2 : Gain  Gain=-1
  Max : MinMax  Function=max  Inputs=2
  Mux : Mux
  Sum2 : Sum  Inputs=|-+
  Sum3 : Sum  Inputs=-+|
  Terminator : Terminator
  Terminator1 : Terminator
  Terminator2 : Terminator
  alpha : Outport
  wires:
  Divide/1 -> Atan/1
  Atan/1 -> Gain2/1
  Gain2/1 -> Mux/4, Mux/2
  Divide1/1 -> Atan1/1
  Atan1/1 -> Sum3/1, Sum2/1
  delta_1/1 -> Sum2/2
  Sum2/1 -> Mux/1
  delta_3/1 -> Sum3/2
  Sum3/1 -> Mux/3
  Mux/1 -> alpha/1
  Vy/1 -> Divide1/2, Divide/2
  Max/1 -> Divide1/1, Divide/1
  Abs/1 -> Max/1
  Abs1/1 -> Max/2
  Vx/1 -> Abs1/1
  Gain/1 -> Abs/1
  Demux/3 -> Terminator/1
  Demux/4 -> Terminator1/1
  Demux/2 -> Terminator2/1
  rho/1 -> Demux/1
  Demux/1 -> Gain/1

== system Car_14DOF_Lat_Long_Control_DATAGEN/Fuerzas/alpha_alt3 ==
  Vx_pp_i : Inport
  Vy_pp_i : Inport  Port=2
  delta_1 : Inport  Port=3
  delta_3 : Inport  Port=4
  Atan{,1..3} (4 alike) : Trigonometry  Operator=atan
  Demux : Demux
  Demux1 : Demux
  Divide{,1..3} (4 alike) : Product  Inputs=*/
  Gain : Gain
  Gain1 : Gain
  Mux : Mux
  Sum1 : Sum  Inputs=-+|
  Sum2 : Sum  Inputs=-+|
  alpha : Outport
  wires:
  Mux/1 -> alpha/1
  Vx_pp_i/1 -> Demux/1
  Vy_pp_i/1 -> Demux1/1
  Demux1/1 -> Divide/1
  Demux/1 -> Divide/2
  Divide/1 -> Atan/1
  delta_1/1 -> Sum2/1
  Sum2/1 -> Mux/1
  Divide1/1 -> Atan1/1
  Gain/1 -> Mux/2
  Demux1/2 -> Divide1/1
  Demux/2 -> Divide1/2
  Divide2/1 -> Atan3/1
  Divide3/1 -> Atan2/1
  Demux1/4 -> Divide2/1
  Demux/4 -> Divide2/2
  Gain1/1 -> Mux/4
  Sum1/1 -> Mux/3
  Demux1/3 -> Divide3/1
  Demux/3 -> Divide3/2
  delta_3/1 -> Sum1/1
  Atan/1 -> Sum2/2
  Atan1/1 -> Gain/1
  Atan2/1 -> Sum1/2
  Atan3/1 -> Gain1/1

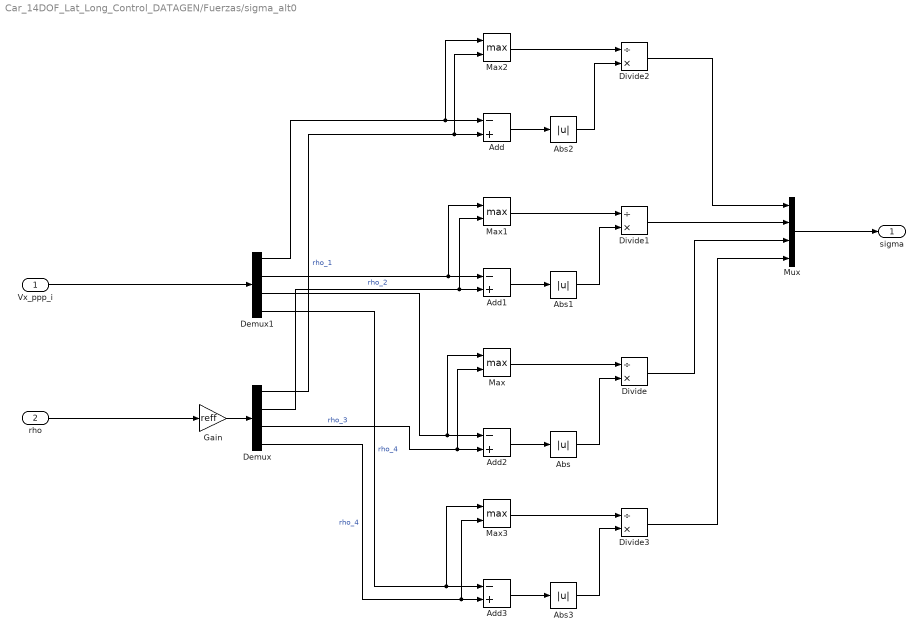
== system Car_14DOF_Lat_Long_Control_DATAGEN/Fuerzas/sigma_alt0 ==
  Vx_ppp_i : Inport
  rho : Inport  Port=2
  Abs{,1..3} (4 alike) : Abs  SaturateOnIntegerOverflow=off
  Add{,1..3} (4 alike) : Sum  Inputs=-+
  Demux : Demux
  Demux1 : Demux
  Divide{,1..3} (4 alike) : Product  Inputs=/*
  Gain : Gain  Gain=reff
  Max{,1..3} (4 alike) : MinMax  Function=max  Inputs=2
  Mux : Mux
  sigma : Outport
  wires:
  Add2/1 -> Abs/1
  Abs/1 -> Divide/2
  Max/1 -> Divide/1
  Add1/1 -> Abs1/1
  Max1/1 -> Divide1/1
  Abs1/1 -> Divide1/2
  Abs2/1 -> Divide2/2
  Add/1 -> Abs2/1
  Max2/1 -> Divide2/1
  Gain/1 -> Demux/1
  Mux/1 -> sigma/1
  rho/1 -> Gain/1
  Vx_ppp_i/1 -> Demux1/1
  Demux/1 -> Max2/2, Add/2  "rho_1"
  Demux1/1 -> Max2/1, Add/1
  Divide2/1 -> Mux/1
  Divide1/1 -> Mux/2
  Demux/2 -> Max1/2, Add1/2  "rho_2"
  Demux1/2 -> Max1/1, Add1/1
  Divide/1 -> Mux/3
  Max3/1 -> Divide3/1
  Add3/1 -> Abs3/1
  Abs3/1 -> Divide3/2
  Divide3/1 -> Mux/4
  Demux/3 -> Max/2, Add2/2  "rho_3"
  Demux1/3 -> Max/1, Add2/1
  Demux/4 -> Max3/2, Add3/2  "rho_4"
  Demux1/4 -> Max3/1, Add3/1  "rho_4"

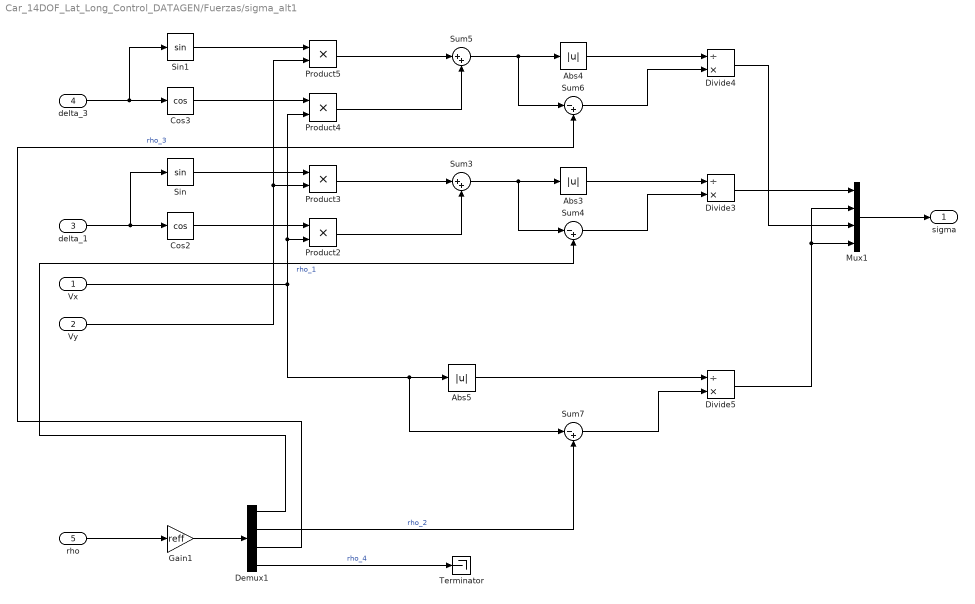
== system Car_14DOF_Lat_Long_Control_DATAGEN/Fuerzas/sigma_alt1 ==
  Vx : Inport
  Vy : Inport  Port=2
  delta_1 : Inport  Port=3
  delta_3 : Inport  Port=4
  rho : Inport  Port=5
  Abs3 : Abs  SaturateOnIntegerOverflow=off
  Abs4 : Abs  SaturateOnIntegerOverflow=off
  Abs5 : Abs  SaturateOnIntegerOverflow=off
  Cos2 : Trigonometry  Operator=cos
  Cos3 : Trigonometry  Operator=cos
  Demux1 : Demux
  Divide3 : Product  Inputs=/*
  Divide4 : Product  Inputs=/*
  Divide5 : Product  Inputs=/*
  Gain1 : Gain  Gain=reff
  Mux1 : Mux
  Product{2..5} (4 alike) : Product
  Sin : Trigonometry
  Sin1 : Trigonometry
  Sum3 : Sum  Inputs=|++
  Sum4 : Sum  Inputs=|-+
  Sum5 : Sum  Inputs=|++
  Sum6 : Sum  Inputs=|-+
  Sum7 : Sum  Inputs=|-+
  Terminator : Terminator
  sigma : Outport
  wires:
  Gain1/1 -> Demux1/1
  Sum5/1 -> Sum6/1, Abs4/1
  Product5/1 -> Sum5/1
  rho/1 -> Gain1/1
  Product3/1 -> Sum3/1
  Demux1/1 -> Sum4/2  "rho_1"
  Demux1/3 -> Sum6/2  "rho_3"
  Sum7/1 -> Divide5/2
  Product2/1 -> Sum3/2
  Abs5/1 -> Divide5/1
  delta_1/1 -> Sin/1, Cos2/1
  Sin/1 -> Product3/1
  delta_3/1 -> Sin1/1, Cos3/1
  Demux1/2 -> Sum7/2  "rho_2"
  Vy/1 -> Product5/2, Product3/2
  Product4/1 -> Sum5/2
  Divide4/1 -> Mux1/3
  Mux1/1 -> sigma/1
  Sum3/1 -> Sum4/1, Abs3/1
  Sum4/1 -> Divide3/2
  Abs3/1 -> Divide3/1
  Abs4/1 -> Divide4/1
  Vx/1 -> Sum7/1, Abs5/1, Product2/2, Product4/2
  Demux1/4 -> Terminator/1  "rho_4"
  Sin1/1 -> Product5/1
  Divide5/1 -> Mux1/2, Mux1/4
  Cos3/1 -> Product4/1
  Sum6/1 -> Divide4/2
  Cos2/1 -> Product2/1
  Divide3/1 -> Mux1/1

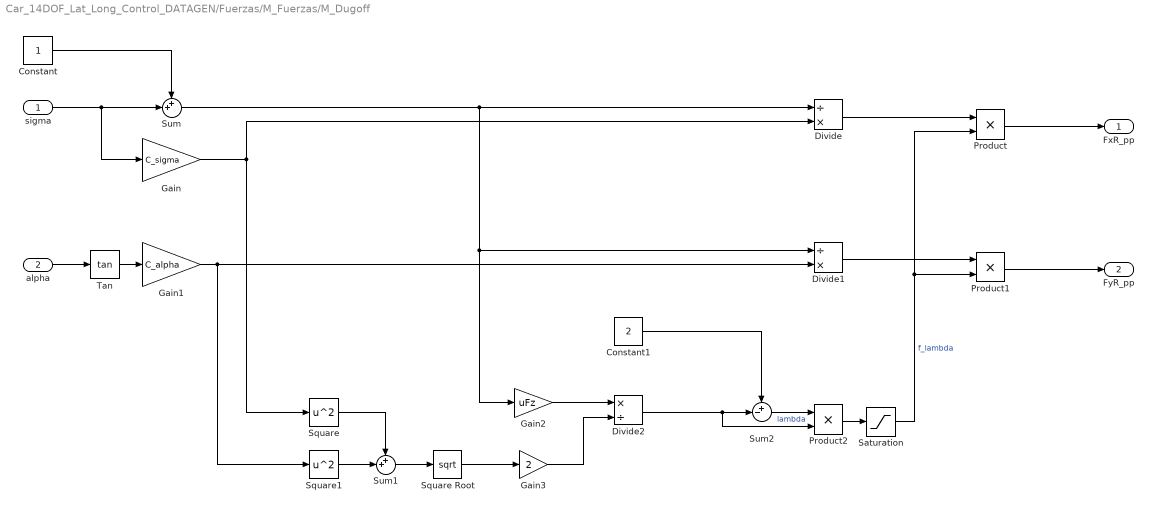
== system Car_14DOF_Lat_Long_Control_DATAGEN/Fuerzas/M_Fuerzas/M_Dugoff ==
  sigma : Inport
  alpha : Inport  Port=2
  Constant : Constant
  Constant1 : Constant  Value=2
  Divide : Product  Inputs=/*
  Divide1 : Product  Inputs=/*
  Divide2 : Product  Inputs=*/
  Gain : Gain  Gain=C_sigma
  Gain1 : Gain  Gain=C_alpha
  Gain2 : Gain  Gain=uFz
  Gain3 : Gain  Gain=2
  Product : Product
  Product1 : Product
  Product2 : Product
  Saturation : Saturate  UpperLimit=1  LowerLimit=-5
  Square : Math  Operator=square
  Square Root : Sqrt
  Square1 : Math  Operator=square
  Sum : Sum  Inputs=++|
  Sum1 : Sum  Inputs=++|
  Sum2 : Sum  Inputs=+-|
  Tan : Trigonometry  Operator=tan
  FxR_pp : Outport
  FyR_pp : Outport  Port=2
  wires:
  alpha/1 -> Tan/1
  sigma/1 -> Gain/1, Sum/2
  Constant/1 -> Sum/1
  Sum/1 -> Divide/1, Divide1/1, Gain2/1
  Gain/1 -> Square/1, Divide/2
  Divide/1 -> Product/1
  Tan/1 -> Gain1/1
  Gain1/1 -> Divide1/2, Square1/1
  Divide1/1 -> Product1/1
  Product/1 -> FxR_pp/1
  Product1/1 -> FyR_pp/1
  Gain2/1 -> Divide2/1
  Square1/1 -> Sum1/2
  Square/1 -> Sum1/1
  Sum1/1 -> Square Root/1
  Gain3/1 -> Divide2/2
  Square Root/1 -> Gain3/1
  Divide2/1 -> Product2/2, Sum2/2  "lambda"
  Constant1/1 -> Sum2/1
  Sum2/1 -> Product2/1
  Product2/1 -> Saturation/1
  Saturation/1 -> Product1/2, Product/2  "f_lambda"

== matlab function Car_14DOF_Lat_Long_Control_DATAGEN/MATLAB Function ==
  settings: updateMethod=DISCRETE
  data: t input; rho_ref output; delta_w output
function [rho_ref, delta_w] = fcn(t)

persistent rho_random randomNumbers;
if isempty(rho_random)
    rng('shuffle'); 
    rho_random = randi([30,150],1,1);
end
rho_ref = rho_random;

%*************************************************
%*************************************************
%*************************************************

% if isempty(randomNumbers)
%     rng('shuffle'); 
%     randomNumbers.randInt1 = randi([-45,45],1,1);
%     randomNumbers.randInt2 = randi([1,10],1,1);
% end
% A = randomNumbers.randInt1;
% b = randomNumbers.randInt2;
% %delta_w = A*sin((2*pi/b)*t);
% %delta_w = A;
% delta_w = A*(1-exp(-t));

if isempty(randomNumbers)
    rng('shuffle'); 
    randomNumbers.randInt1 = randi([-45,45],1,1);
    randomNumbers.randInt2 = randi([-45,45],1,1);
    randomNumbers.randInt3 = randi([-45,45],1,1);
    randomNumbers.randInt4 = randi([-45,45],1,1);
    randomNumbers.randInt5 = randi([2,4],1,1);
    randomNumbers.randInt6 = randi([5,7],1,1);
    randomNumbers.randInt7 = randi([8,9],1,1);
    % randomNumbers.randInt5 = randi([2,5],1,1);
    % randomNumbers.randInt6 = randi([6,9],1,1);
end
y1 = randomNumbers.randInt1;
y2 = randomNumbers.randInt2;
y3 = randomNumbers.randInt3;
y4 = randomNumbers.randInt4;
t2 = randomNumbers.randInt5;
t3 = randomNumbers.randInt6;
t4 = randomNumbers.randInt7;
S = 0;
if t < t2
    S = y1/(1+exp(-10*(t-1)));
end
if t2 <= t && t<t3
    S = y1+(y2-y1)/(1+exp(-10*(t-t2-1)));
end
if t3 <= t && t<t4 %t3<=t 
    S = y2+(y3-y2)/(1+exp(-10*(t-t3-1)));
end
if t >= t4
    S = y3+(y4-y3)/(1+exp(-10*(t-t4-1)));
end
delta_w = S;
